simulink library "cbobsv2"  (Simulink 5.0)
values from neighbouring files (symbols this model uses):
  b = findobj(a, 'Name', get_param(gcbh,'Name'))    [eyesampl2.m]
undefined symbols (not defined in the file or in its folder): eyesampl2
libraries: dspsigattribs x4, dspbuff3 x1
settings Model: Creator=mclune  LastModifiedBy=ysong  ExtModeAutoUpdateStatusClock=off

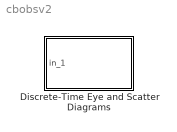
== system cbobsv2 ==
  Discrete-Time Eye and Scatter Diagrams : Subsystem  LoadFcn=eyesampl2([],[],[],'LoadBlock')  StartFcn=eyesampl2([],[],[],'Start')  StopFcn=eyesampl2([],[],[],'Stop')  mask(Discrete-Time Eye and Scatter Diagrams){time_range=1, time_offset=0, time_decision=.5, boundary=[-1.5 1.5], kept_length=5, diagram_type=Eye Diagram, eye_line=b-/r-, scatter_line=b., sample_time=1/100}
      mask prompts: time_range "Trace period:"; time_offset "Trace offset:"; time_decision "Decision point:"; boundary "Lower and upper bounds of diagram (2-element vector):"; kept_length "Number of saved traces:"; diagram_type "Diagram type:"; eye_line "Line type for eye diagram:"; scatter_line "Line type for scatter diagram:"; sample_time "Sample time for plot update:"
      mask help: Create an eye diagram and/or scatter plot, depending on the Diagram type parameter.
      mask init:
      | x = [2 8 5 2 8 5 5 5];
      | y = [2 8 5 8 2 5 8 2];
      | [eStr outparams] = commblkeyescatdisc(gcb,'init');
      | if(eStr .ecode ~= 0)
      |    error(eStr .emsg);
      | end
      settings: CopyFcn=eyesampl2([],[],[],'CopyBlock')  DeleteFcn=eyesampl2([],[],[],'DeleteBlock')  NameChangeFcn=eyesampl2([],[],[],'NameChange')
      mask Help: helpview(commbhelp)
      mask StyleString: edit,edit,edit,edit,edit,popup(Eye Diagram|Scatter Diagram|Eye and Scatter Diagrams),edit,edit,edit
      mask CallbackString: |||||commblkeyescatdisc(gcb,'cbDiagram_type');|||
      mask Display: plot(0,0,100,100,[5 45 45 5 5 5 5+40*[0:1/15:1] 5+40*[1:-1/15:0] 5+40*[0:1/15:1] 5+40*[1:-1/15:0]], [35 35 95 95 35 65 sin([0:1/15:1]*pi)*25+65 sin(-[0:1/15:1]*pi)*25+65 sin([0:1/15:1]*pi)*17+65 sin(-[0:1/15:1]*pi)*18+65] , NaN, NaN, x+50,y+37,x+50,y+52,x+50,y+67,x+50,y+82, x+62,y+37,x+62,y+52,x+62,y+67,x+62,y+82, x+73,y+37,x+73,y+52,x+73,y+67,x+73,y+82, x+85,y+37,x+85,y+52,x+85,y+67,x+85,y+82, [50 95 73 73 73],[65 65 65 35 95])

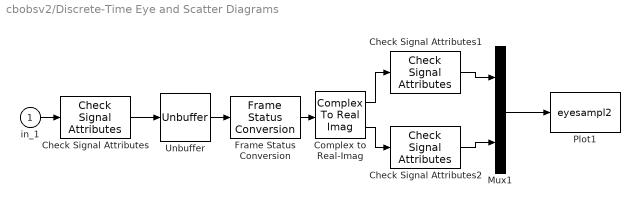
== system cbobsv2/Discrete-Time Eye and Scatter Diagrams ==
  in_1 : Inport
  Check Signal Attributes : dspsigattribs/Check Signal Attributes  SigAttribCheckMethod=Does not match attributes exactly  Complexity=Ignore  Frame=Ignore  DimsCheckMethod=Is...  Dimensions=Column vector (2-D) or scalar  DatatypeCheckMethod=Is not...  DatatypeGeneral=Boolean  DtypeFloatSpecific=Any floating-point  DtypeFixedSpecific=Any fixed-point  DtypeIntSpecific=Any integer  SampleMode=Discrete
  Check Signal Attributes1 : dspsigattribs/Check Signal Attributes  SigAttribCheckMethod=Does not match attributes exactly  Complexity=Ignore  Frame=Ignore  DimsCheckMethod=Is...  Dimensions=Scalar (1-D or 2-D)  DatatypeCheckMethod=Ignore  DatatypeGeneral=Boolean  DtypeFloatSpecific=Any floating-point  DtypeFixedSpecific=Any fixed-point  DtypeIntSpecific=Any integer  SampleMode=Discrete
  Check Signal Attributes2 : dspsigattribs/Check Signal Attributes  SigAttribCheckMethod=Does not match attributes exactly  Complexity=Ignore  Frame=Ignore  DimsCheckMethod=Is...  Dimensions=Scalar (1-D or 2-D)  DatatypeCheckMethod=Ignore  DatatypeGeneral=Boolean  DtypeFloatSpecific=Any floating-point  DtypeFixedSpecific=Any fixed-point  DtypeIntSpecific=Any integer  SampleMode=Discrete
  Complex to Real-Imag : ComplexToRealImag
  Frame Status Conversion : dspsigattribs/Frame Status Conversion  growRefPort=off  outframe=Sample-based
  Mux1 : Mux  Inputs=2
  Plot1 : S-Function  FunctionName=eyesampl2  Parameters=time_range, time_offset, time_decision, boundary, kept_length, diagram_type, eye_line, scatter_line, sample_time
  Unbuffer : dspbuff3/Unbuffer  ic=0
  wires:
  Check Signal Attributes2/1 -> Mux1/2
  Check Signal Attributes1/1 -> Mux1/1
  Frame Status Conversion/1 -> Complex to Real-Imag/1
  Mux1/1 -> Plot1/1
  Complex to Real-Imag/2 -> Check Signal Attributes2/1
  Complex to Real-Imag/1 -> Check Signal Attributes1/1
  in_1/1 -> Check Signal Attributes/1
  Unbuffer/1 -> Frame Status Conversion/1
  Check Signal Attributes/1 -> Unbuffer/1
